simulink model "MassSpringDamper"  (R2017a)
settings: Solver=VariableStepAuto  StartTime=0.0  StopTime=10.0  RelTol=1e-3
model workspace (MAT data in the model file):
  C = 0.84
  F = 4.928
  K = 3.07391304348
  M = 1
libraries: cstblocks x1
settings Model: Creator=gabrieleserra  LastModifiedBy=gabrieleserra

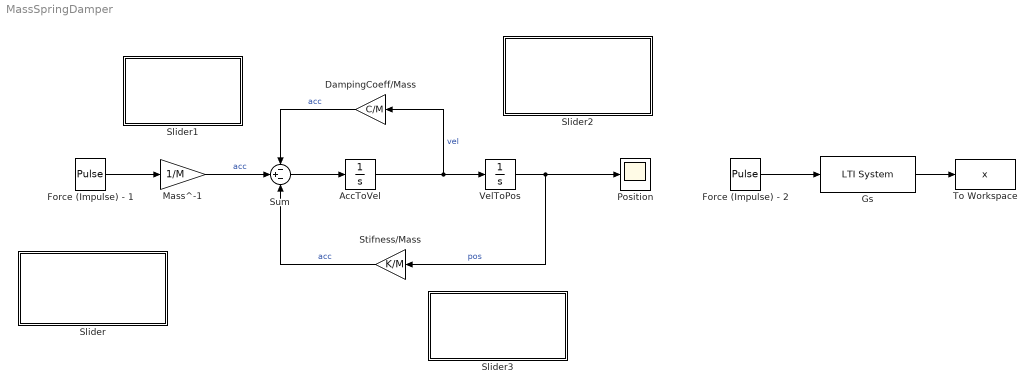
== system MassSpringDamper ==
  AccToVel : Integrator
  DampingCoeff/Mass : Gain  Gain=C/M
  Force (Impulse) - 1 : DiscretePulseGenerator  PulseType=Time based  Amplitude=F  Period=10  PulseWidth=5  PhaseDelay=2
  Force (Impulse) - 2 : DiscretePulseGenerator  PulseType=Time based  Amplitude=F  Period=10  PulseWidth=5  PhaseDelay=2
  Gs : cstblocks/LTI System  sys=tf(1,[M C K])  IC=[]
  Mass^-1 : Gain  Gain=1/M
  Position : Scope
      settings: StopFcn=massspringdamper
  Slider : Subsystem  DialogController=hmiCreateDDGDialog  IsWebBlock=on  mask(MWDashboardBlock){webBlockId=a5e4a0f6-52db-4167-b57c-7df5b6c83942, webBlockType=slider, ShowInLibBrowser=on, ShowInitialText=on, HMISrcModelName=MassSpringDamper}
      mask prompts: webBlockId "WebBlock Id"; webBlockType "WebBlock Type"; HMISrcModelName "Source Model"
      mask help: SimulinkHMI:dialogs:SliderDialogDesc
      mask Help: helpview([docroot '/mapfiles/simulink.map'], 'hmi_slider')
      mask Display:
      | if strcmp(get_param(bdroot(gcb),'BlockDiagramType'), 'library')
      |     image([(matlabroot) '/toolbox/simulink/hmi/icons/Slider.png']);
      | end
  Slider1 : Subsystem  DialogController=hmiCreateDDGDialog  IsWebBlock=on  mask(MWDashboardBlock){webBlockId=e2f55b32-c8e4-48d0-b34b-7f7a50c60807, webBlockType=slider, ShowInLibBrowser=on, ShowInitialText=on, HMISrcModelName=MassSpringDamper}
      mask prompts: webBlockId "WebBlock Id"; webBlockType "WebBlock Type"; HMISrcModelName "Source Model"
      mask help: SimulinkHMI:dialogs:SliderDialogDesc
      mask Help: helpview([docroot '/mapfiles/simulink.map'], 'hmi_slider')
      mask Display:
      | if strcmp(get_param(bdroot(gcb),'BlockDiagramType'), 'library')
      |     image([(matlabroot) '/toolbox/simulink/hmi/icons/Slider.png']);
      | end
  Slider2 : Subsystem  DialogController=hmiCreateDDGDialog  IsWebBlock=on  mask(MWDashboardBlock){webBlockId=a4fb0f92-91dc-4a46-b1d3-3fcb3492cbeb, webBlockType=slider, ShowInLibBrowser=on, ShowInitialText=on, HMISrcModelName=MassSpringDamper}
      mask prompts: webBlockId "WebBlock Id"; webBlockType "WebBlock Type"; HMISrcModelName "Source Model"
      mask help: SimulinkHMI:dialogs:SliderDialogDesc
      mask Help: helpview([docroot '/mapfiles/simulink.map'], 'hmi_slider')
      mask Display:
      | if strcmp(get_param(bdroot(gcb),'BlockDiagramType'), 'library')
      |     image([(matlabroot) '/toolbox/simulink/hmi/icons/Slider.png']);
      | end
  Slider3 : Subsystem  DialogController=hmiCreateDDGDialog  IsWebBlock=on  mask(MWDashboardBlock){webBlockId=a92d69e9-18d5-48ad-8497-0e9b1f4d8810, webBlockType=slider, ShowInLibBrowser=on, ShowInitialText=on, HMISrcModelName=MassSpringDamper}
      mask prompts: webBlockId "WebBlock Id"; webBlockType "WebBlock Type"; HMISrcModelName "Source Model"
      mask help: SimulinkHMI:dialogs:SliderDialogDesc
      mask Help: helpview([docroot '/mapfiles/simulink.map'], 'hmi_slider')
      mask Display:
      | if strcmp(get_param(bdroot(gcb),'BlockDiagramType'), 'library')
      |     image([(matlabroot) '/toolbox/simulink/hmi/icons/Slider.png']);
      | end
  Stifness/Mass : Gain  Gain=K/M
  Sum : Sum  Inputs=-+-
  To Workspace : ToWorkspace  VariableName=x  SaveFormat=Timeseries  SampleTime=-1
  VelToPos : Integrator
  wires:
  Mass^-1/1 -> Sum/2  "acc"
  Sum/1 -> AccToVel/1
  AccToVel/1 -> DampingCoeff/Mass/1, VelToPos/1  "vel"
  VelToPos/1 -> Position/1, Stifness/Mass/1  "pos"
  Stifness/Mass/1 -> Sum/3  "acc"
  DampingCoeff/Mass/1 -> Sum/1  "acc"
  Gs/1 -> To Workspace/1
  Force (Impulse) - 1/1 -> Mass^-1/1
  Force (Impulse) - 2/1 -> Gs/1

== system MassSpringDamper/Slider ==

== system MassSpringDamper/Slider1 ==

== system MassSpringDamper/Slider2 ==

== system MassSpringDamper/Slider3 ==
